simulink model "DC_2_AC_1"  (Simulink 7.4)
settings: Solver=ode23tb  StartTime=0.0  StopTime=1  FixedStep=Ts  RelTol=1e-3  AbsTol=1e-3
PreLoadFcn:
  | assignin('base','Ts',[20e-6])
undefined symbols (not defined in the file or in its folder): Ts
libraries: powerlib x12, powerlib_extras x5, dspsnks4 x3, dspbuff3 x1, dspsigops x1, dspspect3 x1, dsparch4 x1
Description:
  | Copyright 2008 The MathWorks(TM), Inc.
settings Model: Creator=sybille  LastModifiedBy=Dick  ExtModeTrigMode=oneshot  ExtModeArmWhenConnect=off  ExtModeAutoUpdateStatusClock=off
settings DataIOCC: LimitDataPoints=off  SaveOutput=off  SaveTime=off  SignalLoggingName=sigsOut
settings OptimizationCC: BlockReduction=off  BooleanDataType=off  InlineInvariantSignals=on  InitFltsAndDblsToZero=on  EfficientMapNaN2IntZero=off
settings DebuggingCC: SaveWithParameterizedLinksMsg=none  CheckExecutionContextPreStartOutputMsg=on  CheckExecutionContextRuntimeOutputMsg=on  SignalResolutionControl=TryResolveAllWithWarning  SolverPrmCheckMsg=none  MultiTaskDSMMsg=warning  MultiTaskCondExecSysMsg=none  StrictBusMsg=None
settings HardwareCC: TargetUnknown=on
settings RTWCC: IncludeERTFirstTime=on
settings GRTTargetCC: TargetFcnLib=ansi_tfl_tmw.mat

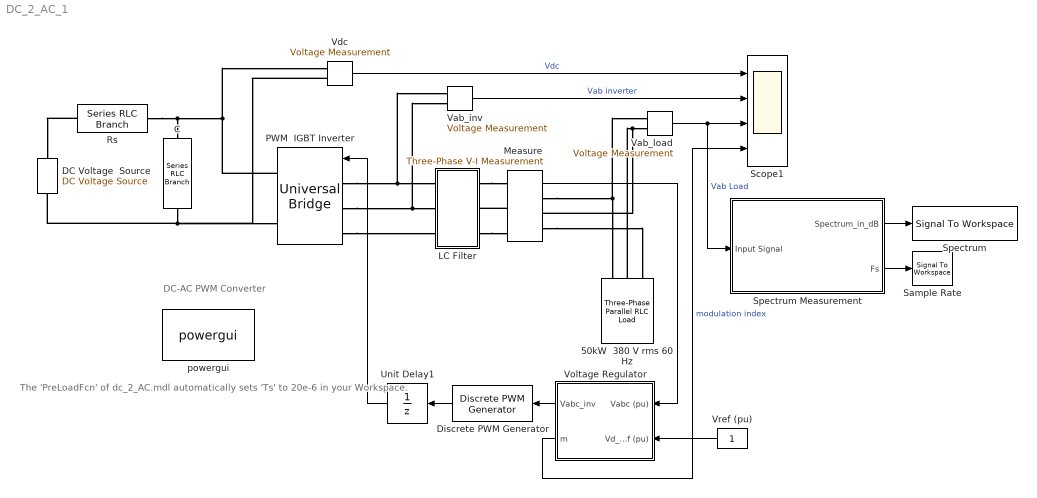
== system DC_2_AC_1 ==
  note: DC-AC PWM Converter
  note: The 'PreLoadFcn' of dc_2_AC.mdl
      | automatically sets 'Ts' to 20e-6 in your Workspace.
  50kW  380 V rms 60 Hz : powerlib/Elements/Three-Phase Parallel RLC Load  DialogController=POWERSYS.PowerSysDialog  PhysicalDomain=powersysdomain  SubClassName=unknown  LeftPortType=p1  RightPortType=p1  LConnTagsString=A|B|C  Configuration=Y (grounded)  NominalVoltage=380  NominalFrequency=60  ActivePower=50e3  InductivePower=0  CapacitivePower=0  Measurements=None
  C : powerlib/Elements/Series RLC Branch  DialogController=POWERSYS.PowerSysDialog  PhysicalDomain=powersysdomain  SubClassName=unknown  LeftPortType=p1  RightPortType=p1  LConnTagsString=__new0  RConnTagsString=__new0  BranchType=C  Resistance=1  Inductance=1e-3  SetiL0=off  InitialCurrent=0  Capacitance=470e-6  Setx0=off  InitialVoltage=0  Measurements=None
  DC Voltage  Source : powerlib/Electrical Sources/DC Voltage Source  DialogController=POWERSYS.PowerSysDialog  SystemSampleTime=-1  Amplitude=sqrt(3)*220*80/38  Measurements=None
  Discrete PWM Generator : powerlib_extras/Discrete  Control Blocks/Discrete PWM Generator  DialogController=POWERSYS.PowerSysDialog  SystemSampleTime=-1  GeneratorMode="3-arm  bridge (6 pulses)"  Fc=2000  Ts=Ts  Internal=off  mIndex=0.4  Freq=60  Phase=0
  LC Filter : Subsystem
  Measure : powerlib/Measurements/Three-Phase V-I Measurement  DialogController=POWERSYS.PowerSysDialog  SystemSampleTime=-1  VoltageMeasurement=phase-to-ground  SetLabelV=off  LabelV=V1  Vpu=on  CurrentMeasurement=no  SetLabelI=off  LabelI=I1  Ipu=off  Pbase=1e3  Vbase=sqrt(3)*220  OutputType=Magnitude  PhasorSimulation=off  PSBequivalent=0
  PWM  IGBT Inverter : powerlib/Power Electronics/Universal Bridge  DialogController=POWERSYS.PowerSysDialog  SystemSampleTime=-1  Arms=3  SnubberResistance=5000  SnubberCapacitance=inf  Device=IGBT / Diodes  Ron=1e-3  Lon=0  ForwardVoltages="[  0.0  0.0  ]"  ForwardVoltage=.8  GTOparameters=[ 1e-6 ,1e-6 ]  IGBTparameters=[ 1e-6 , 2e-6 ]  Measurements=None  Measurements_2=None  converterType=Rectifier
  Rs : powerlib/Elements/Series RLC Branch  DialogController=POWERSYS.PowerSysDialog  PhysicalDomain=powersysdomain  SubClassName=unknown  LeftPortType=p1  RightPortType=p1  LConnTagsString=__new0  RConnTagsString=__new0  BranchType=R  Resistance=.25  Inductance=1e-3  SetiL0=off  InitialCurrent=0  Capacitance=1e-6  Setx0=off  InitialVoltage=0  Measurements=None
  Sample Rate : dspsnks4/Signal To Workspace  SystemSampleTime=-1  VariableName=Fs  FrameMode=Concatenate frames (2-D array)
      settings: MaxDataPoints=1  FixptAsFi=off
  Scope1 : Scope  NumInputPorts=4
      settings: TimeRange=0.1  YMin=600~-1000~-1000~0.4  YMax=900~1000~1000~1  SaveName=psbbridges_str  Decimation=10
  Spectrum : dspsnks4/Signal To Workspace  SystemSampleTime=-1  VariableName=spectrum_dB  FrameMode=Concatenate frames (2-D array)
      settings: MaxDataPoints=1  FixptAsFi=off
  Spectrum Measurement : Subsystem  Description=Spectrum Analyzer  mask{BW=300, Navg=1, Frame=256, Ymin=-20, Ymax=50}
      mask prompts: BW "Bandwidth"; Navg "Number of Averages"; Frame "Frame Size"; Ymin "Ymin_dB"; Ymax "Ymax_dB"
      mask Display: fprintf('Baseband Spectrum Analyzer \n  BW=%7.2f', BW)
  Unit Delay1 : UnitDelay  SampleTime=Ts
  Vab_inv : powerlib/Measurements/Voltage Measurement  Tag=PoWeRsYsTeMmEaSuReMeNt  DialogController=POWERSYS.PowerSysDialog  SystemSampleTime=-1  PhasorSimulation=off  OutputType=Magnitude  PSBequivalent=0
  Vab_load : powerlib/Measurements/Voltage Measurement  Tag=PoWeRsYsTeMmEaSuReMeNt  DialogController=POWERSYS.PowerSysDialog  SystemSampleTime=-1  PhasorSimulation=off  OutputType=Magnitude  PSBequivalent=0
  Vdc : powerlib/Measurements/Voltage Measurement  Tag=PoWeRsYsTeMmEaSuReMeNt  DialogController=POWERSYS.PowerSysDialog  SystemSampleTime=-1  PhasorSimulation=off  OutputType=Magnitude  PSBequivalent=0
  Voltage Regulator : Subsystem  mask( Voltage Regulator){Kp=0.4, Ki=500, Ts=Ts}
      mask prompts: Kp "Proportional gain  Kp:"; Ki "Integral gain Ki:"; Ts "Sample time (s) :"
  "Vref (pu) " : Constant  OutDataType=sfix(16)  OutScaling=2^0
  powergui : powerlib/powergui  Priority=2  SystemSampleTime=-1  SimulationMode=Continuous  SampleTime=Ts  frequency=60  SPID=off  DisableSnubberDevices=off  DisableRonSwitches=off  DisableVfSwitches=off  SwTol=0  Interpol=off  frequencyindice=0  echomessages=on  HookPort=off  DisplayEquations=off  FunctionMessages=off  EnableUseOfTLC=off  x0status=blocks  RestoreLinks=warning  Frange=[0:2:500]  Ylog=off  Xlog=on  ShowGrid=off  save=off  variable=ZData  structure=psbbridges_str  ZoomFFT=on  StartTime=0.1-2/50  cycles=2  DisplayStyle=off  fundamental=50  FreqAxis=off  MaxFrequency=7000  frequencyindicesteady=1  RmsSteady=1  display=off  Ts=0  methode=off
  wires:
  "Vref (pu) "/1 -> Voltage Regulator/2(Vd_ref (pu))
  Discrete PWM Generator/1 -> Unit Delay1/1
  Voltage Regulator/1(Vabc_inv) -> Discrete PWM Generator/1
  Voltage Regulator/2(m) -> Scope1/4  "modulation index"
  Vdc/1 -> Scope1/1  "Vdc"
  Vab_load/1 -> Scope1/3, Spectrum Measurement/1(Input Signal)  "Vab Load"
  Vab_inv/1 -> Scope1/2  "Vab inverter"
  Unit Delay1/1 -> PWM  IGBT Inverter/1
  Measure/1 -> Voltage Regulator/1(Vabc (pu))
  Spectrum Measurement/1(Spectrum_in_dB) -> Spectrum/1
  Spectrum Measurement/2(Fs) -> Sample Rate/1
  connections:
  Vdc/LConn2 -- PWM  IGBT Inverter/RConn2 -- DC Voltage  Source/LConn1 -- C/RConn1
  Rs/RConn1 -- PWM  IGBT Inverter/RConn1 -- Vdc/LConn1 -- C/LConn1
  LC Filter/RConn1 -- Measure/LConn1
  Measure/LConn2 -- LC Filter/RConn2
  LC Filter/RConn3 -- Measure/LConn3
  PWM  IGBT Inverter/LConn2 -- LC Filter/LConn2 -- Vab_inv/LConn2
  PWM  IGBT Inverter/LConn3 -- LC Filter/LConn3
  PWM  IGBT Inverter/LConn1 -- LC Filter/LConn1 -- Vab_inv/LConn1
  Vab_load/LConn2 -- 50kW  380 V rms 60 Hz/LConn2 -- Measure/RConn2
  Measure/RConn1 -- 50kW  380 V rms 60 Hz/LConn1 -- Vab_load/LConn1
  Measure/RConn3 -- 50kW  380 V rms 60 Hz/LConn3
  Rs/LConn1 -- DC Voltage  Source/RConn1

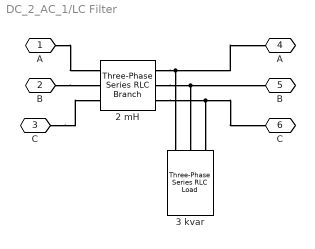
== system DC_2_AC_1/LC Filter ==
  "2 mH " : powerlib/Elements/Three-Phase Series RLC Branch  DialogController=POWERSYS.PowerSysDialog  PhysicalDomain=powersysdomain  SubClassName=unknown  LeftPortType=p1  RightPortType=p1  LConnTagsString=A|B|C  RConnTagsString=A|B|C  BranchType=L  Resistance=1.0  Inductance=2e-3  Capacitance=1.0  Measurements=None
  3 kvar : powerlib/Elements/Three-Phase Series RLC Load  DialogController=POWERSYS.PowerSysDialog  PhysicalDomain=powersysdomain  SubClassName=unknown  LeftPortType=p1  RightPortType=p1  LConnTagsString=A|B|C  Configuration=Y (grounded)  NominalVoltage=380  NominalFrequency=50  ActivePower=0  InductivePower=0  CapacitivePower=3e3  Measurements=None
  A : PMIOPort  Port=1  Side=Left
  B : PMIOPort  Port=2  Side=Left
  C : PMIOPort  Port=3  Side=Left
  "A " : PMIOPort  Port=4  Side=Right
  "B " : PMIOPort  Port=5  Side=Right
  "C " : PMIOPort  Port=6  Side=Right
  connections:
  B/RConn1 -- "2 mH "/LConn2
  A/RConn1 -- "2 mH "/LConn1
  C/RConn1 -- "2 mH "/LConn3
  "2 mH "/RConn1 -- "A "/RConn1 -- 3 kvar/LConn1
  "2 mH "/RConn2 -- "B "/RConn1 -- 3 kvar/LConn2
  "2 mH "/RConn3 -- "C "/RConn1 -- 3 kvar/LConn3

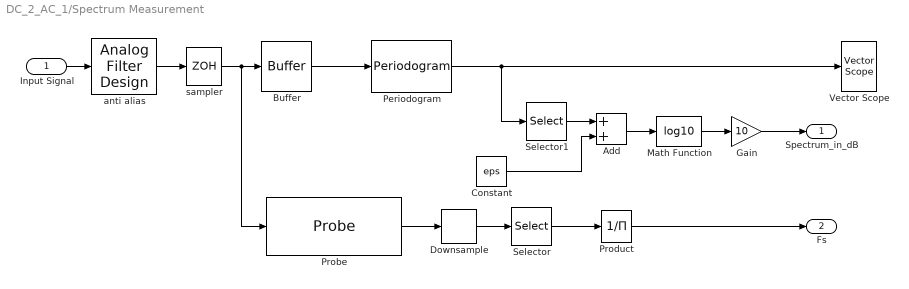
== system DC_2_AC_1/Spectrum Measurement ==
  Input Signal : Inport  OutDataType=sfix(16)  OutScaling=2^0
  Add : Sum  OutDataType=fixdt(1, 16)  OutScaling=2^-10
  Buffer : dspbuff3/Buffer  N=Frame  V=0  ic=0
  Constant : Constant  Value=eps  OutDataType=fixdt(1, 16)  OutScaling=2^0
  Downsample : dspsigops/Downsample  N=Frame  phase=0  ic=0  smode=Allow multirate  fmode=Maintain input frame size
  Gain : Gain  Gain=10  ParameterDataType=fixdt(1, 16)  ParameterScaling=2^0  OutDataType=fixdt(1, 16)  OutScaling=2^0
  Math Function : Math  Operator=log10  OutDataType=fixdt(1, 16)  OutScaling=2^0  SaturateOnIntegerOverflow=on
  Periodogram : dspspect3/Periodogram  SystemSampleTime=-1  measurement=Mean-square spectrum  wintype=Hann  Rs=50  beta=5  winsamp=Symmetric  inheritFFT=on  fftsize=512  navg=Navg  inheritTs=on  Ts=1
  Probe : Probe  ProbeWidth=off  ProbeComplexSignal=off
  Product : Product  Inputs=/  OutDataType=fixdt(1, 16)  OutScaling=2^0  RndMeth=Zero
  Selector : Selector  InputPortWidth=2  IndexOptions=Index vector (dialog)  Indices=1  OutputSizes=1
  Selector1 : Selector  InputPortWidth=Frame  IndexOptions=Index vector (dialog)  Indices=1:Frame/2  OutputSizes=1
  Vector Scope : dspsnks4/Vector Scope  DialogController=dspdialog.VectorScope  DialogControllerArgs=DataTag0  ScopeProperties=on  Domain=Frequency  HorizSpan=1  DisplayProperties=off  AxisGrid=on  Memory=off  FrameNumber=on  AxisLegend=off  AxisZoom=off  OpenScopeAtSimStart=on  OpenScopeImmediately=off  FigPos=[330 35 414 221]  AxisProperties=off  XUnits=Hertz  XRange=[0...Fs/2]  InheritXIncr=on  XIncr=1  XLabel=Time  XLimit=Auto  XMin=0  XMax=1  XStart=0  YUnits=dB  YLabel=dB  LineProperties=off  XAxisParamsVer=6.9
      settings: YMin=Ymin  YMax=Ymax
  anti alias : dsparch4/Analog Filter Design  method=Elliptic  filttype=Lowpass  N=8  Wlo=BW*2*pi  Whi=80  Rp=0.11  Rs=100
  sampler : ZeroOrderHold  SampleTime=1/(2.56*BW)
  Spectrum_in_dB : Outport  OutDataType=fixdt(1, 16)  OutScaling=2^0
  Fs : Outport  Port=2  OutDataType=fixdt(1, 16)  OutScaling=2^0
  wires:
  anti alias/1 -> sampler/1
  Input Signal/1 -> anti alias/1
  sampler/1 -> Buffer/1, Probe/1
  Periodogram/1 -> Vector Scope/1, Selector1/1
  Buffer/1 -> Periodogram/1
  Math Function/1 -> Gain/1
  Gain/1 -> Spectrum_in_dB/1
  Probe/1 -> Downsample/1
  Selector/1 -> Product/1
  Product/1 -> Fs/1
  Downsample/1 -> Selector/1
  Selector1/1 -> Add/1
  Add/1 -> Math Function/1
  Constant/1 -> Add/2

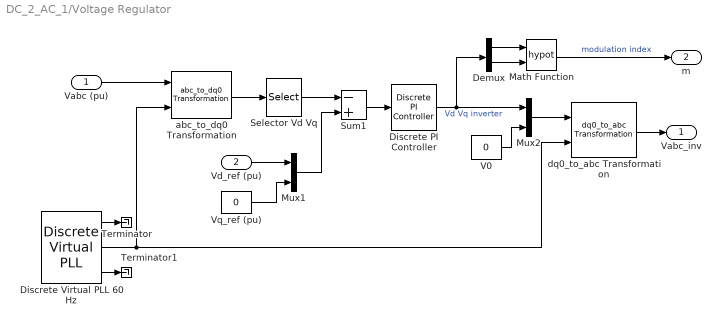
== system DC_2_AC_1/Voltage Regulator ==
  Vabc (pu) : Inport  OutDataType=sfix(16)  OutScaling=2^0
  Vd_ref (pu) : Inport  Port=2  OutDataType=sfix(16)  OutScaling=2^0
  Demux : Demux  Outputs=2
  Discrete PI Controller : powerlib_extras/Discrete  Control Blocks/Discrete PI Controller  DialogController=POWERSYS.PowerSysDialog  SystemSampleTime=-1  Kp=Kp  Ki=Ki  Par_Limits=[1 -1]  Init=0  Ts=Ts
  Discrete Virtual PLL 60 Hz : powerlib_extras/Discrete  Control Blocks/Discrete Virtual PLL  DialogController=POWERSYS.PowerSysDialog  SystemSampleTime=-1  Freq=60  Phase=0  Ts=Ts
  Math Function : Math  Operator=hypot  OutDataType=sfix(16)  OutScaling=2^0  SaturateOnIntegerOverflow=on
  Mux1 : Mux  Inputs=2
  Mux2 : Mux  Inputs=2
  Selector Vd Vq : Selector  InputPortWidth=3  IndexOptions=Index vector (dialog)  Indices=[1 2]  OutputSizes=1
  Sum1 : Sum  Inputs=-+  OutDataType=sfix(16)  OutScaling=2^0  SaturateOnIntegerOverflow=on  InputSameDT=on  OutDataTypeStr=Inherit: Same as first input
  Terminator : Terminator
  Terminator1 : Terminator
  V0 : Constant  Value=0  OutDataType=sfix(16)  OutScaling=2^0
  Vq_ref (pu) : Constant  Value=0  OutDataType=sfix(16)  OutScaling=2^0
  abc_to_dq0 Transformation : powerlib_extras/Measurements/abc_to_dq0 Transformation  DialogController=POWERSYS.PowerSysDialog  SystemSampleTime=-1
  dq0_to_abc Transformation : powerlib_extras/Measurements/dq0_to_abc Transformation  DialogController=POWERSYS.PowerSysDialog  SystemSampleTime=-1
  Vabc_inv : Outport  OutDataType=sfix(16)  OutScaling=2^0
  m : Outport  Port=2  OutDataType=sfix(16)  OutScaling=2^0
  wires:
  abc_to_dq0 Transformation/1 -> Selector Vd Vq/1
  Vabc (pu)/1 -> abc_to_dq0 Transformation/1
  Selector Vd Vq/1 -> Sum1/1
  Sum1/1 -> Discrete PI Controller/1
  Mux2/1 -> dq0_to_abc Transformation/1
  V0/1 -> Mux2/2
  dq0_to_abc Transformation/1 -> Vabc_inv/1
  Discrete Virtual PLL 60 Hz/2 -> abc_to_dq0 Transformation/2, dq0_to_abc Transformation/2
  Vd_ref (pu)/1 -> Mux1/1
  Vq_ref (pu)/1 -> Mux1/2
  Mux1/1 -> Sum1/2
  Discrete Virtual PLL 60 Hz/1 -> Terminator/1
  Discrete Virtual PLL 60 Hz/3 -> Terminator1/1
  Discrete PI Controller/1 -> Demux/1, Mux2/1  "Vd Vq inverter"
  Demux/1 -> Math Function/1
  Demux/2 -> Math Function/2
  Math Function/1 -> m/1  "modulation index"
